simulink model "rester"  (R2016b)
settings: Solver=FixedStepAuto  StartTime=0.0  StopTime=inf  RelTol=1e-3
libraries: embdlinuxlib x1
settings Model: SimulationMode=external  Creator=sbuadu  LastModifiedBy=sbuadu
settings SolverCC: PositivePriorityOrder=on
settings OptimizationCC: MaxStackSize=64
settings DebuggingCC: ParameterTunabilityLossMsg=error
settings HardwareCC: ProdBitPerPointer=32  ProdBitPerSizeT=32  ProdBitPerPtrDiffT=32  ProdLargestAtomicInteger=Long  ProdLargestAtomicFloat=Double  ProdWordSize=32  ProdHWDeviceType=ARM Compatible->ARM Cortex
settings RTWCC: SystemTargetFile=ert.tlc  HardwareBoard=Raspberry Pi  TLCOptions="-aInlineSetEventsForThisBaseRateFcn=TLC_FALSE -aSuppressMultiTaskScheduler=TLC_FALSE  -aRateBasedStepFcn=0"  TemplateMakefile=ert_default_tmf  Description=Embedded Coder  GenerateReport=on  Toolchain=GNU GCC Raspberry Pi  IncludeHyperlinkInReport=on  LaunchReport=on  GenerateTraceInfo=on  GenerateTraceReport=on  GenerateTraceReportSl=on  GenerateTraceReportSf=on  GenerateTraceReportEml=on
settings CodeAppCC: ForceParamTrailComments=on  IgnoreCustomStorageClasses=off  OperatorAnnotations=on  SimulinkDataObjDesc=on  SFDataObjDesc=on  MATLABFcnDesc=on  InsertBlockDesc=on  MATLABSourceComments=on
settings ERTTargetCC: SupportVariableSizeSignals=on

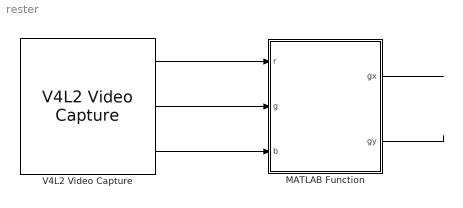
== system rester ==
  MATLAB Function : MATLAB Function  TreatAsAtomicUnit=on
  V4L2 Video Capture : embdlinuxlib/V4L2 Video Capture  m_devName='/dev/video0'  roi=[0, 0, 640, 480]  imSizeSelection=640x480  imSize=[640, 480]  pixelFormat=RGB  pixelOrder=Planar  sampleTime=1  simOutput=Colorbars  blockPlatform=Raspberry Pi
  wires:
  V4L2 Video Capture/2 -> MATLAB Function/2(g)
  V4L2 Video Capture/1 -> MATLAB Function/1(r)
  V4L2 Video Capture/3 -> MATLAB Function/3(b)
  MATLAB Function/1(gx) -> ?
  MATLAB Function/2(gy) -> ?

== matlab function rester/MATLAB Function ==
  data: r input; g input; b input; gx output; gy output
function [gx, gy] = fcn(r,g, b)
image = uint8(zeros(480,640, 3));

image(:,:,1) = r'; 
image(:,:, 2) = g'; 
image(:, :, 3) = b'; 

coder.extrinsic('imshow'); 
imshow(image);
%viscircles(s.Centroid, 10);
%[i,j]=find(greenBinary == 1)


end
